simulink model "test"  (R2016a)
settings: Solver=FixedStepAuto  StartTime=0.0  StopTime=inf  FixedStep=.01  RelTol=1e-3
libraries: LibrarySimulinkSAS x4, visionsinks x3, instrumentlib x2, dspnetwork x1
settings Model: Creator=DSANTIAGO  LastModifiedBy=santd

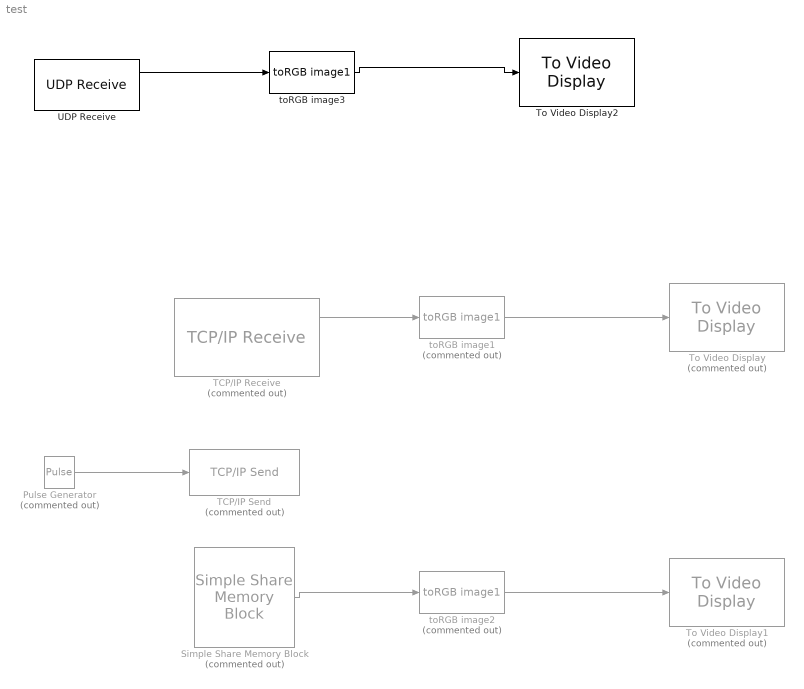
== system test ==
  Pulse Generator : DiscretePulseGenerator  Commented=on  PulseType=Time based  Period=.01  PulseWidth=5
  Simple Share Memory Block : LibrarySimulinkSAS/Simple Share Memory Block  Commented=on  nombre='baseName_output'  dispositivo=1  vecE=[]  vecS=[230400]  tipoE=[]  tipoS=['C']
  TCP/IP Receive : instrumentlib/TCP//IP Receive  Commented=on  Host=190.124.230.171  Port=1234  DataSize=230400  EnableBlockingMode=off  Timeout=10  SampleTime=0.01  DataType=uint8  ByteOrder=BigEndian
  TCP/IP Send : instrumentlib/TCP//IP Send  Commented=on  Host=190.124.230.171  Port=1234  EnableBlockingMode=off  Timeout=10  ByteOrder=BigEndian
  To Video Display : visionsinks/To Video Display  Commented=on  windowSizeMode=Normal  openAtMdlStart=on  fullScreen=off  videoWindowX=536805376  videoWindowY=536805376  saveWindowSize=off  videoWindowWidth=116  videoWindowHeight=64  inputColorFormat=RGB  inputType=Obsolete  imagePorts=One multidimensional signal  OutputDevice=On-screen video monitor  dataOrg=Column-major  isWindowOpen=off
  To Video Display1 : visionsinks/To Video Display  Commented=on  windowSizeMode=Normal  openAtMdlStart=on  fullScreen=off  videoWindowX=536805376  videoWindowY=536805376  saveWindowSize=off  videoWindowWidth=320  videoWindowHeight=240  inputColorFormat=RGB  inputType=Obsolete  imagePorts=One multidimensional signal  OutputDevice=On-screen video monitor  dataOrg=Column-major  isWindowOpen=off
  To Video Display2 : visionsinks/To Video Display  windowSizeMode=Normal  openAtMdlStart=on  fullScreen=off  videoWindowX=536805376  videoWindowY=536805376  saveWindowSize=off  videoWindowWidth=116  videoWindowHeight=64  inputColorFormat=RGB  inputType=Obsolete  imagePorts=One multidimensional signal  OutputDevice=On-screen video monitor  dataOrg=Column-major  isWindowOpen=off
  UDP Receive : dspnetwork/UDP Receive  localURL='0.0.0.0'  localPort=45454  remoteURL='0.0.0.0'  remotePort=-1  recvBufferSize=44100  dims=44100  signalDatatype=uint8  isVarSize=off  showBlockingTime=off  blockingTime=0  sampletime=1
  toRGB image1 : LibrarySimulinkSAS/V-REP Camera/toRGB image1  Commented=on  ResX=320  ResY=240
  toRGB image2 : LibrarySimulinkSAS/V-REP Camera/toRGB image1  Commented=on  ResX=320  ResY=240
  toRGB image3 : LibrarySimulinkSAS/V-REP Camera/toRGB image1  ResX=105  ResY=140
  wires:
  toRGB image1/1 -> To Video Display/1
  TCP/IP Receive/1 -> toRGB image1/1
  Pulse Generator/1 -> TCP/IP Send/1
  Simple Share Memory Block/1 -> toRGB image2/1
  toRGB image2/1 -> To Video Display1/1
  toRGB image3/1 -> To Video Display2/1
  UDP Receive/1 -> toRGB image3/1
